simulink model "LKAS_AutoSave_DF_20220407_0926_SW62"  (R2018b)
settings: Solver=FixedStepDiscrete  StartTime=0.0  StopTime=10.0  FixedStep=0.01  RelTol=1e-3
InitFcn:
  | tmpVer = ver('MATLAB');
  | tmpVer = str2num(tmpVer.Version);
  | % -------------------------------------------------------------------
  | %  MATLAB file generated by Simulink.saveVars on 21-Nov-2019 10:06:14
  | %  MATLAB version: 7.13.0.564 (R2011b)
  | % -------------------------------------------------------------------
  | 
  | 
  | SInt16 = Simulink.AliasType;
  | SInt16.Description = 'Num';
  | if (tmpVer > 7.11)
  | 	SInt16.DataScope = 'Auto';
  | end
  | SInt16.HeaderFile = 'Rte_Type.h';
  | SInt16.BaseType = 'int16';
  | 
  | SInt32 = Simulink.AliasType;
  | SInt32.Description = 'Num';
  | if (tmpVer > 7.11)
  | 	SInt32.DataScope = 'Auto';
  | end
  | SInt32.HeaderFile = 'Rte_Type.h';
  | SInt32.BaseType = 'int32';
  | 
  | SInt8 = Simulink.AliasType;
  | SInt8.Description = 'Num';
  | if (tmpVer > 7.11)
  | 	SInt8.DataScope = 'Auto';
  | end
  | SInt8.HeaderFile = 'Rte_Type.h';
  | SInt8.BaseType = 'int8';
  | 
  | T_A_m2_1024_1_u32 = Simulink.NumericType;
  | T_A_m2_1024_1_u32.Description = 'm2 (square meters  (m2))';
  | if (tmpVer > 7.11)
  | 	T_A_m2_1024_1_u32.DataScope = 'Auto';
  | end
  | T_A_m2_1024_1_u32.HeaderFile = 'Rte_Type.h';
  | T_A_m2_1024_1_u32.DataTypeMode = 'Fixed-point: slope and bias scaling';
  | T_A_m2_1024_1_u32.SignednessBool = false;
  | T_A_m2_1024_1_u32.WordLength = 32;
  | T_A_m2_1024_1_u32.FixedExponent = -10;
  | T_A_m2_1024_1_u32.SlopeAdjustmentFactor = 1;
  | T_A_m2_1024_1_u32.Bias = 0;
  | T_A_m2_1024_1_u32.DataTypeOverride = 'Inherit';
  | T_A_m2_1024_1_u32.IsAlias = true;
  | 
  | T_A_m2_65536_1_u16 = Simulink.NumericType;
  | T_A_m2_65536_1_u16.Description = 'm2 (square meters  (m2))';
  | if (tmpVer > 7.11)
  | 	T_A_m2_65536_1_u16.DataScope = 'Auto';
  | end
  | T_A_m2_65536_1_u16.HeaderFile = 'Rte_Type.h';
  | T_A_m2_65536_1_u16.DataTypeMode = 'Fixed-point: slope and bias scaling';
  | T_A_m2_65536_1_u16.SignednessBool = false;
  | T_A_m2_65536_1_u16.WordLength = 16;
  | T_A_m2_65536_1_u16.FixedExponent = -16;
  | T_A_m2_65536_1_u16.SlopeAdjustmentFactor = 1;
  | T_A_m2_65536_1_u16.Bias = 0;
  | T_A_m2_65536_1_u16.DataTypeOverride = 'Inherit';
  | ... (+4664 lines)
StopFcn:
  | clear  T_A_m2_1024_1_u32 T_A_m2_65536_1_u16 T_A_m2_Float32 T_A_mm2_10_1_u16 T_A_mm2_4_1_s16 T_A_mm2_Float32 T_Cnt_Num_10_1_u32 T_Cnt_Num_1_1_s16 T_Cnt_Num_1_1_s32 T_Cnt_Num_1_1_s8 T_Cnt_Num_1_1_u16 T_Cnt_Num_1_1_u32 T_Cnt_Num_1_1_u8 T_E_J_1_1_s32 T_E_J_Float32 T_E_kJ_128_1_s32 T_E_kJ_Float32 T_E_kwh_10_1_u16 T_E_kwh_Float32 T_Epl_kwhpkm_100_1_u16 T_Epl_kwhpkm_Float32 T_F_N_1_1_s16 T_F_N_Float32 T_I_A_1000_1_u16 T_I_A_1048576_1_s32 T_I_A_2048_1_s16 T_I_A_32_1_s16 T_I_A_Float32 T_I_mA_1_1_s16 T_I_mA_32768_128_s16 T_I_mA_Float32 T_J_kgpm2_128_1_u16 T_J_kgpm2_Float32 T_K_NA_1000_1_s16 T_K_NA_100_1_s16 T_K_NA_100_1_u16 T_K_NA_1024_1_s16 T_K_NA_1024_1_u16 T_K_NA_128_1_s16 T_K_NA_128_1_u16 T_K_NA_128_1_u8 T_K_NA_16777216_1_u32 T_K_NA_16_1_s16 T_K_NA_16_1_u16 T_K_NA_16_1_u8 T_K_NA_1_16_u16 T_K_NA_1_1_s16 T_K_NA_1_1_u16 T_K_NA_1_1_u8 T_K_NA_32768_1_s16 T_K_NA_32768_1_u16 T_K_NA_32_1_s8 T_K_NA_4096_1_u16 T_K_NA_4194304_1_s32 T_K_NA_4194304_1_u16 T_K_NA_65536_1_s32 T_K_NA_65536_1_u16 T_K_NA_8192_1_s16 T_K_NA_8_1_s16 T_K_NA_Float32 T_M_Nm_16_1_s16 T_M_Nm_1_1_s16 T_M_Nm_32768_1_s16 T_M_Nm_32_1_s16 T_M_Nm_4_1_s16 T_M_Nm_512_1_s16 T_M_Nm_Float32 T_P_W_1_4_s16 T_P_W_1_8_s16 T_P_W_Float32 T_P_kW_128_1_s16 T_P_kW_1_8_s16 T_P_kW_8_1_s32 T_P_kW_Float32 T_Pct_pct_1024_1_s32 T_Pct_pct_1024_1_u32 T_Pct_pct_10_1_s16 T_Pct_pct_10_1_u32 T_Pct_pct_128_100_s8 T_Pct_pct_1_1_s16 T_Pct_pct_1_4_u8 T_Pct_pct_255_100_u16 T_Pct_pct_255_100_u8 T_Pct_pct_256_1_s16 T_Pct_pct_256_1_u16 T_Pct_pct_65535_100_u16 T_Pct_pct_Float32 T_R_ohm_1024_1_s16 T_R_ohm_32_1_s16 T_R_ohm_Float32 T_TK_K_16_1_s16 T_TK_K_Float32 T_T_degC_10_400_1_u16 T_T_degC_16_1_s16 T_T_degC_1_40_1_u8 T_T_degC_2_80_1_u8 T_T_degC_Float32 T_U_V_1000_1_u16 T_U_V_10_1_u8 T_U_V_200_1_u8 T_U_V_32_1_s16 T_U_V_4096_1_s16 T_U_V_512_1_s16 T_U_V_65535_8_u16 T_U_V_8192_1_u16 T_U_V_Float32 T_U_mV_1_1_s16 T_U_mV_256_20_u16 T_U_mV_Float32 T_V_l_256_1_s16 T_V_l_4096_1_s16 T_V_l_64_1_s16 T_V_l_65535_100_u16 T_V_l_Float32 T_V_ml_128_1_s16 T_V_ml_1_1_s16 T_V_ml_32768_1_s16 T_V_ml_Float32 T_V_ul_32_1_u16 T_V_ul_Float32 T_Vpl_clpkm_512_1_u16 T_Vpl_clpkm_Float32 T_a_kphps_16_1_s16 T_a_kphps_Float32 T_a_mps2_128_1_s16 T_a_mps2_Float32 T_c_MJpkg_256_1_s16 T_c_MJpkg_Float32 T_c_kJpgpK_1024_1_s16 T_c_kJpgpK_Float32 T_c_kJpkgpK_128_1_u16 T_c_kJpkgpK_Float32 T_chrg_Ah_1_1_s16 T_chrg_Ah_1_1_u16 T_chrg_Ah_1_1_u8 T_chrg_Ah_256_1_u16 T_chrg_Ah_4194304_1_s32 T_chrg_Ah_512_1_u16 T_chrg_Ah_8_1_u16 T_chrg_Ah_Float32 T_cmp_NA_100_1_s16 T_cmp_NA_128_1_s16 T_cmp_NA_16_1_s16 T_cmp_NA_32768_1_u16 T_cmp_NA_Float32 T_d2n_rpmps2_4_1_s16 T_d2n_rpmps2_Float32 T_dPct_pctps_16_1_s16 T_dPct_pctps_256_1_s16 T_dPct_pctps_Float32 T_dT_degCps_128_1_s16 T_dT_degCps_Float32 T_dV_lph_1_1_s16 T_dV_lph_Float32 T_dV_lpm_128_1_s16 T_dV_lpm_32_1_s16 T_dV_lpm_Float32 T_dV_lps_1024_1_u16 T_dV_lps_4_1_u16 T_dV_lps_Float32 T_dV_mlps_1024_1_s16 T_dV_mlps_Float32 T_d_BitField16 T_dm_gps_128_1_s16 T_dm_gps_128_1_u16 T_dm_gps_256_1_u16 T_dm_gps_Float32 T_dm_mgps_1_1_s16 T_dm_mgps_Float32 T_dn_rpmps_1_1_s16 T_dn_rpmps_2_1_s16 T_dn_rpmps_Float32 T_dp_Paps_1_1_s16 T_dp_Paps_Float32 T_dp_kPaps_1_1_s16 T_dp_kPaps_8_1_s16 T_dp_kPaps_Float32 T_dphi_degps_128_1_s16 T_dphi_degps_8_1_s16 T_dphi_degps_Float32 T_dr_ps_256_1_s16 T_dr_ps_Float32 T_drho_mgplps_1_2_s16 T_drho_mgplps_Float32 T_e_NA_1_1_u8 T_f_Hz_1_1_u16 T_f_Hz_1_1_u32 T_f_Hz_64_1_u16 T_f_Hz_8_1_s16 T_f_Hz_Float32 T_g_BitField32 T_l_km_16_1_s16 T_l_km_1_1_u16 T_l_km_1_1_u32 T_l_km_Float32 T_l_m_1024_1_s16 T_l_m_16_1_s16 T_l_m_1_1_u32 T_l_m_Float32 T_l_mm_16_1_s16 T_l_mm_1_1_u16 T_l_mm_4096_1_s16 T_l_mm_4_1_u8 T_l_mm_64_1_s16 T_l_mm_Float32 T_m_g_1_1_s16 T_m_g_2048_1_s16 T_m_g_32_1_u16 T_m_g_Float32 T_m_kg_1024_1_s16 T_m_kg_1_1_s16 T_m_kg_1_1_u32 T_m_kg_Float32 T_m_mg_128_1_s16 T_m_mg_32_1_s16 T_m_mg_Float32 T_n_rpm_1_1_s16 T_n_rpm_1_25_u8 T_n_rpm_256_50_u16 T_n_rpm_2_25_u8 T_n_rpm_4_1_u16 T_n_rpm_Float32 T_p_MPa_64_1_s16 T_p_MPa_Float32 T_p_Pa_1_1_s16 T_p_Pa_Float32 T_p_kPa_1_10_u16 T_p_kPa_1_1_s16 T_p_kPa_1_1_u8 T_p_kPa_256_1_u16 T_p_kPa_32_1_u16 T_p_kPa_64_1_s16 T_p_kPa_Float32 T_phi_deg_100_1_s16 T_phi_deg_1024_1_s16 T_phi_deg_128_1_s16 T_phi_deg_1_1_u8 T_phi_deg_256_1_s16 T_phi_deg_2_1_s8 T_phi_deg_32_1_s16 T_phi_deg_512_6_s32 T_phi_deg_Float32 T_phi_rad_2048_1_s16 T_phi_rad_Float32 T_r_NA_1024_1_s16 T_r_NA_1024_1_u16 T_r_NA_16384_1_s16 T_r_NA_16_1_s16 T_r_NA_256_1_s8 T_r_NA_256_1_u16 T_r_NA_32768_1_u16 T_r_NA_32_1_u16 T_r_NA_4096_1_s16 T_r_NA_65535_2_u16 T_r_NA_8192_1_u16 T_r_NA_Float32 T_rho_gpl_8192_1_s16 T_rho_gpl_Float32 T_rho_kgpm3_16_1_s16 T_rho_kgpm3_Float32 T_rho_mgpl_1_1_s16 T_rho_mgpl_64_1_s16 T_rho_mgpl_Float32 T_t_hour_1_1_s16 T_t_hour_Float32 T_t_m_1_1_u16 T_t_m_Float32 T_t_ms_1_1_s16 T_t_ms_1_1_u16 T_t_ms_1_1_u32 T_t_ms_4096_1_s16 T_t_ms_64_1_s16 T_t_ms_Float32 T_t_s_1000_1_s16 T_t_s_100_1_s16 T_t_s_10_1_s16 T_t_s_10_1_u16 T_t_s_1_1_s16 T_t_s_1_1_u16 T_t_s_1_1_u32 T_t_s_Float32 T_t_us_10_1_u32 T_t_us_1_1_s16 T_t_us_1_1_u32 T_t_us_1_4_u16 T_t_us_Float32 T_v_kph_1_1_u8 T_v_kph_64_1_s16 T_v_kph_64_1_u16 T_v_kph_Float32 T_v_mps_256_1_s16 T_v_mps_Float32 T_w_radps_32_1_s16 T_w_radps_Float32 T_y_BitField8 T_y_BitFieldDiagProgress T_y_BitFieldDiagStatus T_y_NA_1_1_u8 SInt16 SInt32 SInt8 T_BOOLEAN UInt16 UInt32 UInt8 s16 s32 s8 u16 u32 u8
model workspace (MAT data in the model file):
  MCOS : class17 (value not decoded)
  MCOS : class17 (value not decoded)
  MCOS : class17 (value not decoded)
  MCOS : class17 (value not decoded)
  MCOS : class17 (value not decoded)
  MCOS : class17 (value not decoded)
  MCOS : class17 (value not decoded)
  MCOS : class17 (value not decoded)
  MCOS : class17 (value not decoded)
  MCOS : class17 (value not decoded)
  MCOS : class17 (value not decoded)
  MCOS : class17 (value not decoded)
  MCOS : class17 (value not decoded)
  MCOS : class17 (value not decoded)
  MCOS : class17 (value not decoded)
  MCOS : class17 (value not decoded)
  MCOS : class17 (value not decoded)
  MCOS : class17 (value not decoded)
  MCOS : class17 (value not decoded)
  MCOS : class17 (value not decoded)
  MCOS : class17 (value not decoded)
  MCOS : class17 (value not decoded)
  MCOS : class17 (value not decoded)
  MCOS : class17 (value not decoded)
  MCOS : class17 (value not decoded)
  MCOS : class17 (value not decoded)
  MCOS : class17 (value not decoded)
  MCOS : class17 (value not decoded)
  MCOS : class17 (value not decoded)
  MCOS : class17 (value not decoded)
  MCOS : class17 (value not decoded)
  MCOS : class17 (value not decoded)
  MCOS : class17 (value not decoded)
  MCOS : class17 (value not decoded)
  MCOS : class17 (value not decoded)
  MCOS : class17 (value not decoded)
  MCOS : class17 (value not decoded)
  MCOS : class17 (value not decoded)
  MCOS : class17 (value not decoded)
  MCOS : class17 (value not decoded)
  MCOS : class17 (value not decoded)
  MCOS : class17 (value not decoded)
  MCOS : class17 (value not decoded)
  MCOS : class17 (value not decoded)
  MCOS : class17 (value not decoded)
  MCOS : class17 (value not decoded)
  MCOS : class17 (value not decoded)
  MCOS : class17 (value not decoded)
  MCOS : class17 (value not decoded)
  MCOS : class17 (value not decoded)
  MCOS : class17 (value not decoded)
  MCOS : class17 (value not decoded)
  MCOS : class17 (value not decoded)
  MCOS : class17 (value not decoded)
  MCOS : class17 (value not decoded)
  MCOS : class17 (value not decoded)
  MCOS : class17 (value not decoded)
  MCOS : class17 (value not decoded)
  MCOS : class17 (value not decoded)
  MCOS : class17 (value not decoded)
  MCOS : class17 (value not decoded)
  MCOS : class17 (value not decoded)
  MCOS : class17 (value not decoded)
  MCOS : class17 (value not decoded)
  MCOS : class17 (value not decoded)
  MCOS : class17 (value not decoded)
  MCOS : class17 (value not decoded)
  MCOS : class17 (value not decoded)
  MCOS : class17 (value not decoded)
  MCOS : class17 (value not decoded)
  MCOS : class17 (value not decoded)
  MCOS : class17 (value not decoded)
  MCOS : class17 (value not decoded)
  MCOS : class17 (value not decoded)
  MCOS : class17 (value not decoded)
  MCOS : class17 (value not decoded)
  MCOS : class17 (value not decoded)
  MCOS : class17 (value not decoded)
  MCOS : class17 (value not decoded)
  MCOS : class17 (value not decoded)
  MCOS : class17 (value not decoded)
  MCOS : class17 (value not decoded)
  MCOS : class17 (value not decoded)
  MCOS : class17 (value not decoded)
  MCOS : class17 (value not decoded)
  MCOS : class17 (value not decoded)
  MCOS : class17 (value not decoded)
  MCOS : class17 (value not decoded)
  MCOS : class17 (value not decoded)
  MCOS : class17 (value not decoded)
  MCOS : class17 (value not decoded)
  MCOS : class17 (value not decoded)
  MCOS : class17 (value not decoded)
  MCOS : class17 (value not decoded)
  MCOS : class17 (value not decoded)
  MCOS : class17 (value not decoded)
  MCOS : class17 (value not decoded)
  MCOS : class17 (value not decoded)
  MCOS : class17 (value not decoded)
  MCOS : class17 (value not decoded)
  MCOS : class17 (value not decoded)
  MCOS : class17 (value not decoded)
  MCOS : class17 (value not decoded)
  MCOS : class17 (value not decoded)
  MCOS : class17 (value not decoded)
  MCOS : class17 (value not decoded)
undefined symbols (not defined in the file): LKA_CarWidth, LKA_SampleTime, LKA_StrRatio_C, LKA_Veh2CamL_C, LKA_Veh2CamW_C, LKA_WhlBaseL_C, LL_CompHdAg_C, LL_CompSWA_C, LL_CrvtPrvwT_C, LL_DesDvt_C, LL_DvtComp_C, LL_DvtPrvwT_C, LL_DvtSpdDet_vDvtSpdMin_C, LL_HandsOff_ExitTime, LL_HandsOff_TextTime, LL_HandsOff_WarnTime, LL_HdAgExT_C, LL_HdAgPrvwT_C, LL_LAccMax_C, LL_LAccRMax_C, LL_LDW_EarliestWarnLine_C, LL_LDW_LatestWarnLine_C, LL_LDWS_SUPPRESS_HEADING, LL_LFClb_TFC_FfCtlRatio_C, LL_LFClb_TFC_KdBalance_C, LL_LFClb_TFC_KdMaxSWA_C, LL_LFClb_TFC_KdV1_C, LL_LFClb_TFC_KdV2_C, LL_LFClb_TFC_KdVehSpdLwr_C, LL_LFClb_TFC_KdVehSpdUpr_C, LL_LFClb_TFC_Ki_C, LL_LFClb_TFC_KiMaxSWA_C, LL_LFClb_TFC_Kp_C, LL_LFClb_TFC_KpKlat_C, LL_LFClb_TFC_KpV1_C, LL_LFClb_TFC_KpV2_C, LL_LFClb_TFC_KpVehSpdLwr_C, LL_LFClb_TFC_KpVehSpdUpr_C, LL_LFClb_TFC_PrvwT_C, LL_LKA_EarliestWarnLine_C, LL_LKA_LatestWarnLine_C, LL_LKAExPrcs_ExitC0Dvt, LL_LKAExPrcs_ExitC0Swt, LL_LKAExPrcs_tiExitDelayTime3, LL_LKAExPrcs_tiExitTime1, LL_LKAExPrcs_tiExitTime2, LL_LKAExPrcs_tiExitTime3, LL_LKAS_OUT_OF_CONTROL_LAT_VEL, LL_LKAS_OUT_OF_CONTROL_TTLC, LL_LKASWASyn_M0, LL_LKASWASyn_M1, LL_LKASWASyn_M2, LL_LKASWASyn_M3D, LL_LKASWASyn_M3K_DT, LL_LKASWASyn_M3K_MSD, LL_LKASWASyn_M4K, LL_LKASWASyn_SWAaddMax, LL_LKASWASyn_T2, LL_LKASWASyn_tiTrqSwaRtTime, LL_LKASWASyn_tiTrqSwaTime ... (+47)
libraries: simulink x234, canmsglib x6, dspstat3 x3, simulink_extras x1
(part 12 of 22)

== system LKAS_AutoSave_DF_20220407_0926_SW62/LKAS/LL/LLOn/LKA Input Processing (LKAInP)/Previewed Heading Angle Calculation (PrHdAg)/Perdicted Heading Angle from Right Lane Line (PrvwTTLCHdAgLftTTLCRgt) ==
  PrdcHdAgRgt_lPrvwDstZ : Inport
  PrdcHdAgRgt_bsR0Info : Inport  Port=2
  Add : Sum  Inputs=+++  AccumDataTypeStr=single
  Bus Selector : BusSelector  OutputSignals=R0_C1,R0_C2,R0_C3
  Gain : Gain  Gain=2  OutDataTypeStr=single
  Gain1 : Gain  Gain=3  OutDataTypeStr=single
  Product3 : Product  OutDataTypeStr=single  RndMeth=Zero
  Product4 : Product  OutDataTypeStr=single  RndMeth=Zero
  Z*Z : Product  OutDataTypeStr=single  RndMeth=Zero
  PrdcHdAgRgt_phiPrdcHdAgRgt : Outport
  wires:
  Add/1 -> PrdcHdAgRgt_phiPrdcHdAgRgt/1
  PrdcHdAgRgt_bsR0Info/1 -> Bus Selector/1
  PrdcHdAgRgt_lPrvwDstZ/1 -> Z*Z/1, Product3/2, Z*Z/2
  Bus Selector/1 -> Add/1  "<R0_C1>"
  Product3/1 -> Add/2
  Bus Selector/2 -> Gain/1  "<R0_C2>"
  Bus Selector/3 -> Gain1/1  "<R0_C3>"
  Product4/1 -> Add/3
  Z*Z/1 -> Product4/2
  Gain/1 -> Product3/1
  Gain1/1 -> Product4/1

== system LKAS_AutoSave_DF_20220407_0926_SW62/LKAS/LL/LLOn/LKA Input Processing (LKAInP)/Previewed Heading Angle Calculation (PrHdAg)/Perdicted Heading Angle from Right Lane Line (PrvwTTLCHdAgRgtTTLCRgt) ==
  PrdcHdAgRgt_lPrvwDstZ : Inport
  PrdcHdAgRgt_bsR0Info : Inport  Port=2
  Add : Sum  Inputs=+++  AccumDataTypeStr=single
  Bus Selector : BusSelector  OutputSignals=R0_C1,R0_C2,R0_C3
  Gain : Gain  Gain=2  OutDataTypeStr=single
  Gain1 : Gain  Gain=3  OutDataTypeStr=single
  Product3 : Product  OutDataTypeStr=single  RndMeth=Zero
  Product4 : Product  OutDataTypeStr=single  RndMeth=Zero
  Z*Z : Product  OutDataTypeStr=single  RndMeth=Zero
  PrdcHdAgRgt_phiPrdcHdAgRgt : Outport
  wires:
  Gain1/1 -> Product4/1
  Gain/1 -> Product3/1
  Z*Z/1 -> Product4/2
  Product4/1 -> Add/3
  Bus Selector/3 -> Gain1/1  "<R0_C3>"
  Bus Selector/2 -> Gain/1  "<R0_C2>"
  Product3/1 -> Add/2
  Bus Selector/1 -> Add/1  "<R0_C1>"
  PrdcHdAgRgt_lPrvwDstZ/1 -> Z*Z/2, Product3/2, Z*Z/1
  PrdcHdAgRgt_bsR0Info/1 -> Bus Selector/1
  Add/1 -> PrdcHdAgRgt_phiPrdcHdAgRgt/1

== system LKAS_AutoSave_DF_20220407_0926_SW62/LKAS/LL/LLOn/LKA Input Processing (LKAInP)/Previewed Heading Angle Calculation (PrHdAg)/Predicted Heading Angle from Left Lane Line (PrdcHdAgtLft)1 ==
  PrdcHdAgtLft_bsL0Info : Inport
  PrdcHdAgtLft_lPrvwDstZ : Inport  Port=2
  Add : Sum  Inputs=+++  AccumDataTypeStr=single
  Bus Selector : BusSelector  OutputSignals=L0_C1,L0_C2,L0_C3
  Gain : Gain  Gain=2  OutDataTypeStr=single
  Gain1 : Gain  Gain=3  OutDataTypeStr=single
  Product3 : Product  OutDataTypeStr=single  RndMeth=Zero
  Product4 : Product  OutDataTypeStr=single  RndMeth=Zero
  Z*Z : Product  OutDataTypeStr=single  RndMeth=Zero
  PrdcHdAgtLft_phiPrdcHdAgLft : Outport
  wires:
  Gain1/1 -> Product4/1
  Gain/1 -> Product3/1
  Z*Z/1 -> Product4/2
  Product4/1 -> Add/3
  Bus Selector/3 -> Gain1/1  "<L0_C3>"
  Bus Selector/2 -> Gain/1  "<L0_C2>"
  Product3/1 -> Add/2
  Bus Selector/1 -> Add/1  "<L0_C1>"
  PrdcHdAgtLft_lPrvwDstZ/1 -> Z*Z/2, Product3/2, Z*Z/1
  PrdcHdAgtLft_bsL0Info/1 -> Bus Selector/1
  Add/1 -> PrdcHdAgtLft_phiPrdcHdAgLft/1

== system LKAS_AutoSave_DF_20220407_0926_SW62/LKAS/LL/LLOn/LKA Input Processing (LKAInP)/Previewed Heading Angle Calculation (PrHdAg)/Predicted Heading Angle from Left Lane Line (PrdcHdAgtLftTTLCLft) ==
  PrdcHdAgtLft_bsL0Info : Inport
  PrdcHdAgtLft_lPrvwDstZ : Inport  Port=2
  Add : Sum  Inputs=+++  AccumDataTypeStr=single
  Bus Selector : BusSelector  OutputSignals=L0_C1,L0_C2,L0_C3
  Gain : Gain  Gain=2  OutDataTypeStr=single
  Gain1 : Gain  Gain=3  OutDataTypeStr=single
  Product3 : Product  OutDataTypeStr=single  RndMeth=Zero
  Product4 : Product  OutDataTypeStr=single  RndMeth=Zero
  Z*Z : Product  OutDataTypeStr=single  RndMeth=Zero
  PrdcHdAgtLft_phiPrdcHdAgLft : Outport
  wires:
  Gain1/1 -> Product4/1
  Gain/1 -> Product3/1
  Z*Z/1 -> Product4/2
  Product4/1 -> Add/3
  Bus Selector/3 -> Gain1/1  "<L0_C3>"
  Bus Selector/2 -> Gain/1  "<L0_C2>"
  Product3/1 -> Add/2
  Bus Selector/1 -> Add/1  "<L0_C1>"
  PrdcHdAgtLft_lPrvwDstZ/1 -> Z*Z/2, Product3/2, Z*Z/1
  PrdcHdAgtLft_bsL0Info/1 -> Bus Selector/1
  Add/1 -> PrdcHdAgtLft_phiPrdcHdAgLft/1

== system LKAS_AutoSave_DF_20220407_0926_SW62/LKAS/LL/LLOn/LKA Input Processing (LKAInP)/Previewed Heading Angle Calculation (PrHdAg)/Predicted Heading Angle from Left Lane Line (PrvwTTLCHdAgRgtTTLCLft) ==
  PrdcHdAgtLft_bsL0Info : Inport
  PrdcHdAgtLft_lPrvwDstZ : Inport  Port=2
  Add : Sum  Inputs=+++  AccumDataTypeStr=single
  Bus Selector : BusSelector  OutputSignals=L0_C1,L0_C2,L0_C3
  Gain : Gain  Gain=2  OutDataTypeStr=single
  Gain1 : Gain  Gain=3  OutDataTypeStr=single
  Product3 : Product  OutDataTypeStr=single  RndMeth=Zero
  Product4 : Product  OutDataTypeStr=single  RndMeth=Zero
  Z*Z : Product  OutDataTypeStr=single  RndMeth=Zero
  PrdcHdAgtLft_phiPrdcHdAgLft : Outport
  wires:
  Add/1 -> PrdcHdAgtLft_phiPrdcHdAgLft/1
  PrdcHdAgtLft_bsL0Info/1 -> Bus Selector/1
  PrdcHdAgtLft_lPrvwDstZ/1 -> Z*Z/1, Product3/2, Z*Z/2
  Bus Selector/1 -> Add/1  "<L0_C1>"
  Product3/1 -> Add/2
  Bus Selector/2 -> Gain/1  "<L0_C2>"
  Bus Selector/3 -> Gain1/1  "<L0_C3>"
  Product4/1 -> Add/3
  Z*Z/1 -> Product4/2
  Gain/1 -> Product3/1
  Gain1/1 -> Product4/1

== system LKAS_AutoSave_DF_20220407_0926_SW62/LKAS/LL/LLOn/LKA Input Processing (LKAInP)/Previewed Heading Angle Calculation (PrHdAg)/Z Calculation (ZCalc) ==
  ZCalc_vVehSpd : Inport
  ZCalc_tiHdAgPrvwT_C : Inport  Port=2
  Divide : Product  Inputs=**  OutDataTypeStr=single
  kph to mps : Gain  Gain=1/3.6  OutDataTypeStr=single
  ZCalc_lPrvwDstZ : Outport
  wires:
  kph to mps/1 -> Divide/1
  Divide/1 -> ZCalc_lPrvwDstZ/1
  ZCalc_tiHdAgPrvwT_C/1 -> Divide/2
  ZCalc_vVehSpd/1 -> kph to mps/1

== system LKAS_AutoSave_DF_20220407_0926_SW62/LKAS/LL/LLOn/LKA Input Processing (LKAInP)/Previewed Heading Angle Calculation (PrHdAg)/Z Calculation (ZCalc)1 ==
  ZCalc_vVehSpd : Inport
  ZCalc_tiHdAgPrvwT_C : Inport  Port=2
  Divide : Product  Inputs=**  OutDataTypeStr=single
  kph to mps : Gain  Gain=1/3.6  OutDataTypeStr=single
  ZCalc_lPrvwDstZ : Outport
  wires:
  kph to mps/1 -> Divide/1
  Divide/1 -> ZCalc_lPrvwDstZ/1
  ZCalc_tiHdAgPrvwT_C/1 -> Divide/2
  ZCalc_vVehSpd/1 -> kph to mps/1

== system LKAS_AutoSave_DF_20220407_0926_SW62/LKAS/LL/LLOn/LKA Input Processing (LKAInP)/Steering Wheel Position Calculation (SWAPosCal)/Subsystem ==
  SWAIn : Inport
  LKA_SampleTime : Inport  Port=2
  Enable : EnablePort
      settings: AttributesFormatString=states = %<StatesWhenEnabling>
  Constant : Constant  Value=10  OutDataTypeStr=single
  LowPass : Subsystem
  Saturation : Saturate  UpperLimit=3  LowerLimit=-3
      settings: AttributesFormatString="Min = %<LowerLimit>  Max = %<UpperLimit>"
  SWAPos : Outport  InitialOutput=0
      settings: AttributesFormatString=%<OutputWhenDisabled> = %<InitialOutput>
  wires:
  SWAIn/1 -> LowPass/2(u)
  LowPass/1(y) -> Saturation/1  "SWAPos"
  Constant/1 -> LowPass/1(T)
  LKA_SampleTime/1 -> LowPass/3(dT)
  Saturation/1 -> SWAPos/1

== system LKAS_AutoSave_DF_20220407_0926_SW62/LKAS/LL/LLOn/LKA Input Processing (LKAInP)/Steering Wheel Position Calculation (SWAPosCal)/Subsystem1 ==
  L0 : Inport
  R0 : Inport  Port=2
  VehSpd : Inport  Port=3
  SWA : Inport  Port=4
  LKA_SampleTime : Inport  Port=5
  Abs{2,4..7} (5 alike) : Abs
  Bus Selector : BusSelector  OutputSignals=L0_C1,L0_C2,L0_Q
  Bus Selector1 : BusSelector  OutputSignals=R0_C1,R0_C2,R0_Q
  Compare To Constant : simulink/Logic and Bit Operations/Compare To Constant  relop===  const=3.0  OutDataTypeStr=boolean
  Compare To Constant1 : simulink/Logic and Bit Operations/Compare To Constant  relop===  const=3.0  OutDataTypeStr=boolean
  Constant : Constant  Value=0.0001  OutDataTypeStr=single
  Constant1 : Constant  Value=0.008  OutDataTypeStr=single
  Constant3 : Constant  Value=2  OutDataTypeStr=single
  Constant4 : Constant  Value=35  OutDataTypeStr=single
  Constant5 : Constant  Value=4  OutDataTypeStr=single
  Divide : Product  Inputs=*/
  Logical Operator : Logic  AllPortsSameDT=off  OutDataTypeStr=boolean
  Logical Operator1 : Logic  AllPortsSameDT=off  OutDataTypeStr=boolean
  Logical Operator3 : Logic  Inputs=5  AllPortsSameDT=off  OutDataTypeStr=boolean
  Logical Operator4 : Logic  AllPortsSameDT=off  OutDataTypeStr=boolean
  Relational Operator{,1..3,7} (5 alike) : RelationalOperator  Operator=<=  OutDataTypeStr=boolean  RndMeth=Simplest
  Relational Operator6 : RelationalOperator  OutDataTypeStr=boolean  RndMeth=Simplest
  Subsystem : Subsystem
  Flg : Outport
  wires:
  L0/1 -> Bus Selector/1
  R0/1 -> Bus Selector1/1
  Logical Operator1/1 -> Logical Operator3/1
  Bus Selector/3 -> Compare To Constant/1  "<L0_Q>"
  Abs2/1 -> Relational Operator7/1
  Bus Selector1/3 -> Compare To Constant1/1  "<R0_Q>"
  Relational Operator2/1 -> Logical Operator1/1
  Compare To Constant1/1 -> Logical Operator4/2
  Relational Operator6/1 -> Logical Operator3/4
  Abs7/1 -> Relational Operator3/1
  Constant1/1 -> Relational Operator3/2, Relational Operator2/2
  Constant/1 -> Relational Operator1/2, Relational Operator/2
  Abs4/1 -> Relational Operator/1
  Constant3/1 -> Divide/1
  Logical Operator3/1 -> Subsystem/Enable, Subsystem/1(In)  "SWA"
  VehSpd/1 -> Relational Operator6/1
  Constant4/1 -> Relational Operator6/2
  Abs6/1 -> Relational Operator2/1
  Compare To Constant/1 -> Logical Operator4/1
  Relational Operator7/1 -> Logical Operator3/5
  Bus Selector1/2 -> Abs5/1  "<R0_C2>"
  Abs5/1 -> Relational Operator1/1
  Relational Operator1/1 -> Logical Operator/2
  Relational Operator3/1 -> Logical Operator1/2
  SWA/1 -> Abs2/1
  Logical Operator/1 -> Logical Operator3/2
  Constant5/1 -> Relational Operator7/2
  Subsystem/1(Out) -> Flg/1
  Bus Selector/1 -> Abs6/1  "<L0_C1>"
  Bus Selector1/1 -> Abs7/1  "<R0_C1>"
  Logical Operator4/1 -> Logical Operator3/3
  Bus Selector/2 -> Abs4/1  "<L0_C2>"
  Divide/1 -> Subsystem/2(In1)
  Relational Operator/1 -> Logical Operator/1
  LKA_SampleTime/1 -> Divide/2

== system LKAS_AutoSave_DF_20220407_0926_SW62/LKAS/LL/LLOn/LKA Input Processing (LKAInP)/Under The Limit (UndrLim)/Steering Wheel Angel Max (SWAMax) ==
  SWAMax_vVehSpd : Inport
  SWAMax_aLAcc_C : Inport  Port=2
  LKA_StrRatio_C : Inport  Port=3
  LKA_WhlBaseL_C : Inport  Port=4
  Constant : Constant  Value=0.09  OutDataTypeStr=single
  Divide1 : Product  Inputs=*/
  MATLAB Function : MATLAB Function  TreatAsAtomicUnit=on
  Saturation1 : Saturate  UpperLimit=0.0117  LowerLimit=0.00237
      settings: AttributesFormatString="Min = %<LowerLimit>  Max = %<UpperLimit>"
  Saturation3 : Saturate  UpperLimit=150  LowerLimit=60
      settings: AttributesFormatString="Min = %<LowerLimit>  Max = %<UpperLimit>"
  kph To mps : Gain  Gain=1/3.6  OutDataTypeStr=single
  SWAMax_phiSWAMax : Outport
  wires:
  LKA_StrRatio_C/1 -> MATLAB Function/3(i)
  LKA_WhlBaseL_C/1 -> MATLAB Function/4(L)
  kph To mps/1 -> MATLAB Function/1(v)
  SWAMax_vVehSpd/1 -> Saturation3/1, kph To mps/1
  Divide1/1 -> Saturation1/1
  Saturation1/1 -> MATLAB Function/5(K)
  SWAMax_aLAcc_C/1 -> MATLAB Function/2(ax)
  MATLAB Function/1(SWAmax) -> SWAMax_phiSWAMax/1
  Constant/1 -> Divide1/1
  Saturation3/1 -> Divide1/2  "Vx"

== system LKAS_AutoSave_DF_20220407_0926_SW62/LKAS/LL/LLOn/LKA Input Processing (LKAInP)/Under The Limit (UndrLim)/Steering Wheel Angel Rate Max (SWARMax) ==
  SWARateMax_vVehSpd : Inport
  SWARateMax_aLAccR_C : Inport  Port=2
  LKA_StrRatio_C : Inport  Port=3
  LKA_WhlBaseL_C : Inport  Port=4
  Constant : Constant  Value=0.09  OutDataTypeStr=single
  Divide1 : Product  Inputs=*/
  MATLAB Function : MATLAB Function  TreatAsAtomicUnit=on
  Saturation1 : Saturate  UpperLimit=0.0117  LowerLimit=0.00237
      settings: AttributesFormatString="Min = %<LowerLimit>  Max = %<UpperLimit>"
  Saturation3 : Saturate  UpperLimit=150  LowerLimit=60
      settings: AttributesFormatString="Min = %<LowerLimit>  Max = %<UpperLimit>"
  kph To mps : Gain  Gain=1/3.6  OutDataTypeStr=single
  SWARMax_dphiSWARMax : Outport
  wires:
  kph To mps/1 -> MATLAB Function/1(v)
  LKA_WhlBaseL_C/1 -> MATLAB Function/4(L)
  LKA_StrRatio_C/1 -> MATLAB Function/3(i)
  MATLAB Function/1(SWARmax) -> SWARMax_dphiSWARMax/1
  SWARateMax_vVehSpd/1 -> Saturation3/1, kph To mps/1
  Divide1/1 -> Saturation1/1
  Saturation1/1 -> MATLAB Function/5(K)
  SWARateMax_aLAccR_C/1 -> MATLAB Function/2(dax)
  Constant/1 -> Divide1/1
  Saturation3/1 -> Divide1/2  "Vx"

== system LKAS_AutoSave_DF_20220407_0926_SW62/LKAS/LL/LLOn/LL State Determination (LLStateDet)/LL State Machine Conditions (LLSMCon)/Activation Condition (ActvC) ==
  LKA_Mode : Inport
  bsInInfo : Inport  Port=2
  bsLKAInPInfo : Inport  Port=3
  bsLLClb : Inport  Port=4
  Activation Condition Synthesis (ActvCSyn) : Subsystem  Description=|
      | Block Name: Activation Condition Synthesis
      | Ab.: ActvCSyn
      | No.: 1.1.1.4.4
      | Rev: 0.0.1
      | Update Date: 19-3-26
  Bus Selector : BusSelector  OutputSignals=bsEPSInfo,bsLaneInfo.bsL0Info.L0_Q,bsLaneInfo.bsR0Info.R0_Q
  Bus Selector1 : BusSelector  OutputSignals=LaneWidth,bsDvtInfo.ILftDvt,bsDvtInfo.IRgtDvt
  Deviation Threshold Condition (DvtThresCon) : Subsystem
  EPS Controllability Enable Condition (EPSCtlEC) : Subsystem  Description=|
      | Block Name: EPS Controllability Enable Condition
      | Ab.: EPSCtlEC
      | No.: 1.1.1.4.1
      | Rev: 0.0.1
      | Update Date: 19-3-26
  Lane Quality Enable Condition (LaneQlEC) : Subsystem  Description=|
      | Block Name: Lane Quality Enable Condition
      | Ab.: LaneQlEC
      | No.: 1.1.1.4.3
      | Rev: 0.0.1
      | Update Date: 19-3-26
  stLDWActvCSyn : Outport
  stLKAActvCSyn : Outport  Port=2
  wires:
  bsInInfo/1 -> Bus Selector/1, Lane Quality Enable Condition (LaneQlEC)/1(LaneQlEC_InInfoSyn)
  Activation Condition Synthesis (ActvCSyn)/1(stLDWActvCSyn) -> stLDWActvCSyn/1  "stLDWActvCSyn"
  Deviation Threshold Condition (DvtThresCon)/2(stDvtThresActvFlgLKA) -> Activation Condition Synthesis (ActvCSyn)/4(stDvtThresActvFlgLKA), Lane Quality Enable Condition (LaneQlEC)/3(LaneQlEC_stDvtThresActvFlg)
  Bus Selector/1 -> EPS Controllability Enable Condition (EPSCtlEC)/1(EPSCtlEC_bsEPSInfo)  "<bsEPSInfo>"
  Bus Selector/2 -> Lane Quality Enable Condition (LaneQlEC)/4(LaneQlEC_stFacmL0Ql)  "<L0_Q>"
  Bus Selector/3 -> Lane Quality Enable Condition (LaneQlEC)/5(LaneQlEC_stFacmR0Ql)  "<R0_Q>"
  EPS Controllability Enable Condition (EPSCtlEC)/1(stEPSCtlEC) -> Activation Condition Synthesis (ActvCSyn)/2(stEPSCtlEC)
  Lane Quality Enable Condition (LaneQlEC)/1(stLaneQlECFlg) -> Activation Condition Synthesis (ActvCSyn)/5(stLaneQlECFlg)
  Activation Condition Synthesis (ActvCSyn)/2(stLKAActvCSyn) -> stLKAActvCSyn/1  "stLKAActvCSyn"
  bsLLClb/1 -> Deviation Threshold Condition (DvtThresCon)/4(DvtThresCon_bsDvtThresClb), Lane Quality Enable Condition (LaneQlEC)/2(LaneQlEC_SingleLane_Disable_Swt)
  Deviation Threshold Condition (DvtThresCon)/1(stDvtThresActvFlgLDW) -> Activation Condition Synthesis (ActvCSyn)/3(stDvtThresActvFlgLDW)
  bsLKAInPInfo/1 -> Bus Selector1/1, Deviation Threshold Condition (DvtThresCon)/5(DvtThresCon_LKAInfoSyn)
  Bus Selector1/2 -> Deviation Threshold Condition (DvtThresCon)/2(DvtThresCon_ILftDvt)  "<ILftDvt>"
  Bus Selector1/3 -> Deviation Threshold Condition (DvtThresCon)/3(DvtThresCon_IRgtDvt)  "<IRgtDvt>"
  Bus Selector1/1 -> Deviation Threshold Condition (DvtThresCon)/1(DvtThresCon_lLaneWidth)  "<LaneWidth>"
  LKA_Mode/1 -> [LKA_Mode]
  [LKA_Mode] -> Activation Condition Synthesis (ActvCSyn)/1(LKA_Mode)

== system LKAS_AutoSave_DF_20220407_0926_SW62/LKAS/LL/LLOn/LL State Determination (LLStateDet)/LL State Machine Conditions (LLSMCon)/Deactivation Condition (DeactvC) ==
  LKA_Mode : Inport
  bsInInfo : Inport  Port=2
  bsLKAInPInfo : Inport  Port=3
  bsLLClb : Inport  Port=4
  LLState : Inport  Port=5
  ExitFlg : Inport  Port=6
  Bus Selector : BusSelector  OutputSignals=bsVehMovInfo.ESC_VehSpd,bsEPSInfo
  Bus Selector1 : BusSelector  OutputSignals=LaneWidth,bsDvtInfo.ILftDvt,bsDvtInfo.IRgtDvt,bsPrCrvtInfo.crPrvwCrvt
  Deactivation Condition Synthesis (DeactvCSyn) : Subsystem  Description=|
      | Block Name: Deactivation Condition Synthesis
      | Ab.: DeactvCSyn
      | No.: 1.1.1.5.3
      | Rev: 0.0.1
      | Update Date: 19-3-26
  Deviation Threshold Condition (DvtThresCon) : Subsystem
  Driver Take Condition (DvrTkCon) : Subsystem  Description=|
      | Block Name: EPS Condition
      | Ab.: EPSC
      | No.: 1.1.1.5.2
      | Rev: 0.0.1
      | Update Date: 19-3-26
  EPS Condition (EPSC) : Subsystem  Description=|
      | Block Name: EPS Condition
      | Ab.: EPSC
      | No.: 1.1.1.5.2
      | Rev: 0.0.1
      | Update Date: 19-3-26
  stLDWDeactvCSyn : Outport
  stLKADeactvCSyn : Outport  Port=2
  wires:
  bsInInfo/1 -> Bus Selector/1
  Deactivation Condition Synthesis (DeactvCSyn)/1(stLDWDeactvCSyn) -> stLDWDeactvCSyn/1
  bsLLClb/1 -> Deviation Threshold Condition (DvtThresCon)/4(LLClb), Driver Take Condition (DvrTkCon)/3(LLClb), EPS Condition (EPSC)/1(LLClb)
  Deviation Threshold Condition (DvtThresCon)/2(stDvtThresActvFlgLKA) -> Deactivation Condition Synthesis (DeactvCSyn)/3(stDvtThresActvFlgLKA), Driver Take Condition (DvrTkCon)/2(DvtThresCon_stDvtThresActvFlgLKA)
  LLState/1 -> EPS Condition (EPSC)/3(LLState)
  Bus Selector/2 -> EPS Condition (EPSC)/2(bsEPSInfo), Driver Take Condition (DvrTkCon)/5(bsEPSInfo)  "<bsEPSInfo>"
  EPS Condition (EPSC)/1(EPSC_stEPSCFlg) -> Deactivation Condition Synthesis (DeactvCSyn)/5(EPSC_stEPSCFlg)
  ExitFlg/1 -> Deactivation Condition Synthesis (DeactvCSyn)/6(ExitFlg)
  LKA_Mode/1 -> Deactivation Condition Synthesis (DeactvCSyn)/1(LKAMode)
  Deactivation Condition Synthesis (DeactvCSyn)/2(stLKADeactvCSyn) -> stLKADeactvCSyn/1  "stLKADeactvCSyn"
  Bus Selector/1 -> Driver Take Condition (DvrTkCon)/4(ESC_VehSpd)  "<ESC_VehSpd>"
  Driver Take Condition (DvrTkCon)/1(stDvrTkConFlg) -> Deactivation Condition Synthesis (DeactvCSyn)/4(stDvrTkConFlg)
  bsLKAInPInfo/1 -> Deviation Threshold Condition (DvtThresCon)/5(LKAInPInfo), Bus Selector1/1
  Bus Selector1/3 -> Deviation Threshold Condition (DvtThresCon)/3(IRgtDvt)  "<IRgtDvt>"
  Bus Selector1/2 -> Deviation Threshold Condition (DvtThresCon)/2(ILftDvt)  "<ILftDvt>"
  Bus Selector1/4 -> Driver Take Condition (DvrTkCon)/1(crPrvwCrvt)  "<crPrvwCrvt>"
  Bus Selector1/1 -> Deviation Threshold Condition (DvtThresCon)/1(LaneWidth)  "<LaneWidth>"
  Deviation Threshold Condition (DvtThresCon)/1(stDvtThresActvFlgLDW) -> Deactivation Condition Synthesis (DeactvCSyn)/2(stDvtThresActvFlgLDW)

== system LKAS_AutoSave_DF_20220407_0926_SW62/LKAS/LL/LLOn/LL State Determination (LLStateDet)/LL State Machine Conditions (LLSMCon)/Disable Condition (DisblC) ==
  LKA_Mode : Inport
  bsInInfo : Inport  Port=2
  bsLKAInPInfo : Inport  Port=3
  bsLLClb : Inport  Port=4
  LLState : Inport  Port=5
  Disable Condition Synthesis (DisblCSyn) : Subsystem  Description=|
      | Block Name: Disable Condition Synthesis
      | Ab.: DisblCSyn
      | No.: 1.1.1.3.8.0
      | Rev: 0.0.1
      | Update Date: 19-3-26
  Driver Intent Condition (DrvInttC) : Subsystem  Description=|
      | Block Name: Driver Intent Condition
      | Ab.: DrvInttC
      | No.: 1.1.1.3.3.0
      | Rev: 0.0.1
      | Update Date: 19-3-26
  LDW Alarm Timeout (LDWAlrmTOut) : Subsystem  Description=|
      | Block Name: LDW Alarm Timeout
      | Ab.: LDWAlrmTOut
      | No.: 1.1.1.3.6.0
      | Rev: 0.0.1
      | Update Date: 19-3-26
  LDW Own Condition (LDWOwnC) : Subsystem  Description=|
      | Block Name: LDW Own Condition
      | Ab.: LDWOwnC
      | No.: 1.1.1.3.4.0
      | Rev: 0.0.1
      | Update Date: 19-3-26
  LKA Own Condition (LKAOwnC) : Subsystem  Description=|
      | Block Name: LKA Own Condition
      | Ab.: LKAOwnC
      | No.: 1.1.1.3.5.0
      | Rev: 0.0.1
      | Update Date: 19-3-26
  Lane Condition (LaneC) : Subsystem  Description=|
      | Block Name: Lane Condition
      | Ab.: LaneC
      | No.: 1.1.1.3.2.0
      | Rev: 0.0.1
      | Update Date: 19-3-26
  Subsystem : Subsystem  Commented=on
  Subsystem1 : Subsystem
  Vehicle State Condition (VehStateC) : Subsystem  Description=|
      | Block Name: Vehicle State Condition
      | Ab.: VehStateC
      | No.: 1.1.1.3.1.0
      | Rev: 0.0.1
      | Update Date: 19-3-26
  stLDWDisblCSyn : Outport
  stLKADisblCSyn : Outport  Port=2
  Disable_Reason : Outport  Port=3
  wires:
  Vehicle State Condition (VehStateC)/1(stVehStateC) -> [stVehStateC]  "stVehStateC"
  LDW Own Condition (LDWOwnC)/1(stLDWOwnC) -> [stLDWOwnC]  "stLDWOwnC"
  Disable Condition Synthesis (DisblCSyn)/1(stLDWDisblCSyn) -> stLDWDisblCSyn/1  "stLDWDisblCSyn"
  LDW Alarm Timeout (LDWAlrmTOut)/1(stLDWAlrmTOut) -> [stLDWAlrmTOut]  "stLDWAlrmTOut"
  Disable Condition Synthesis (DisblCSyn)/2(stLKADisblCSyn) -> stLKADisblCSyn/1  "stLKADisblCSyn"
  LKA Own Condition (LKAOwnC)/2(LKAOwnCSyn) -> [LKAOwnCSyn]  "LKAOwnCSyn"
  Driver Intent Condition (DrvInttC)/2(DrvInttCSyn) -> [DrvInttCSyn]  "DrvInttCSyn"
  Lane Condition (LaneC)/2(LaneCSyn) -> [LaneCSyn]  "LaneCSyn"
  Vehicle State Condition (VehStateC)/2(VehStateC) -> [VehStateC]  "VehStateC"
  Subsystem1/1(DisableReason) -> Disable_Reason/1  "Disable_Reason"
  LKA_Mode/1 -> [LKA_Mode]
  [LKA_Mode] -> Disable Condition Synthesis (DisblCSyn)/1(LKA_Mode)  "LKA_Mode"
  [LKA_Mode] -> Vehicle State Condition (VehStateC)/1(LKA_Mode)  "LKA_Mode"
  [LKA_Mode] -> LDW Own Condition (LDWOwnC)/1(LKA_Mode)  "LKA_Mode"
  [LKA_Mode] -> LKA Own Condition (LKAOwnC)/1(LKA_Mode)  "LKA_Mode"
  Lane Condition (LaneC)/1(stLaneC) -> [stLaneC]  "stLaneC"
  Driver Intent Condition (DrvInttC)/1(stDrvInttC) -> [stDrvInttC]  "stDrvInttC"
  LKA Own Condition (LKAOwnC)/1(stLKAOwnC) -> [stLKAOwnC]  "stLKAOwnC"
  [stVehStateC] -> Disable Condition Synthesis (DisblCSyn)/2(stVehStateC)
  [stLaneC] -> Disable Condition Synthesis (DisblCSyn)/3(stLaneC)
  [stDrvInttC] -> Disable Condition Synthesis (DisblCSyn)/4(stDrvInttC)
  [stLKAOwnC] -> Disable Condition Synthesis (DisblCSyn)/7(stLKAOwnC)
  [stLDWOwnC] -> Disable Condition Synthesis (DisblCSyn)/5(stLDWOwnC)
  [stLDWAlrmTOut] -> Disable Condition Synthesis (DisblCSyn)/6(stLDWAlrmTOut)
  LDW Alarm Timeout (LDWAlrmTOut)/2(LDWAlrmTOutSyn) -> [LDWAlrmTOutSyn]  "LDWAlrmTOutSyn"
  [LDWAlrmTOutSyn] -> Subsystem1/6(LDWAlrmTOut)
  [DrvInttCSyn] -> Subsystem1/3(DrvInttCSyn)
  [LDWOwnCSyn] -> Subsystem1/4(LDWOwnCSyn)
  [LKAOwnCSyn] -> Subsystem1/5(LKAOwnCSyn)
  [LaneCSyn] -> Subsystem1/2(LaneCSyn)
  [VehStateC] -> Subsystem1/1(VehStateC)
  bsLLClb/1 -> [LLClb]
  [LLClb] -> Vehicle State Condition (VehStateC)/3(LLClb)  "LLClb"
  [LLClb] -> Lane Condition (LaneC)/3(LLClb)  "LLClb"
  [LLClb] -> Driver Intent Condition (DrvInttC)/2(DrvInttC_bsLLClb)  "LLClb"
  [LLClb] -> LDW Own Condition (LDWOwnC)/3(LLClb)  "LLClb"
  [LLClb] -> LKA Own Condition (LKAOwnC)/5(LLClb)  "LLClb"
  [LLClb] -> LDW Alarm Timeout (LDWAlrmTOut)/2(LDWAlrmTOut_bsLLClb)
  LLState/1 -> [LLState]
  [LLState] -> Vehicle State Condition (VehStateC)/4(LLState)  "LLState"
  [LLState] -> LKA Own Condition (LKAOwnC)/4(LLState)  "LLState"
  [LLState] -> LDW Alarm Timeout (LDWAlrmTOut)/1(LDWAlrmTOut_bsLLState)
  bsInInfo/1 -> [InInfoSyn]
  [InInfoSyn] -> Vehicle State Condition (VehStateC)/2(InInfoSyn)  "InInfoSyn"
  [InInfoSyn] -> Lane Condition (LaneC)/1(InInfoSyn)  "InInfoSyn"
  [InInfoSyn] -> Driver Intent Condition (DrvInttC)/1(DrvInttC_bsInInfoSyn)  "InInfoSyn"
  [InInfoSyn] -> LKA Own Condition (LKAOwnC)/2(InInfoSyn)  "InInfoSyn"
  bsLKAInPInfo/1 -> [LKAInPInfo]
  [LKAInPInfo] -> Lane Condition (LaneC)/2(LKAInPInfo)  "LKAInPInfo"
  [LKAInPInfo] -> Driver Intent Condition (DrvInttC)/3(LKAInPInfo)  "LKAInPInfo"
  [LKAInPInfo] -> LDW Own Condition (LDWOwnC)/2(LKAInPInfo)  "LKAInPInfo"
  [LKAInPInfo] -> LKA Own Condition (LKAOwnC)/3(LKAInPInfo)  "LKAInPInfo"
  LDW Own Condition (LDWOwnC)/2(LDWOwnCSyn) -> [LDWOwnCSyn]  "LDWOwnCSyn"

== system LKAS_AutoSave_DF_20220407_0926_SW62/LKAS/LL/LLOn/LL State Determination (LLStateDet)/LL State Machine Conditions (LLSMCon)/Enable Condition (EnaC) ==
  LKA_Mode : Inport
  bsInInfo : Inport  Port=2
  bsLKAInPInfo : Inport  Port=3
  bsLLClb : Inport  Port=4
  Driver Intent Condition (DrvInttC) : Subsystem  Description=|
      | Block Name: Driver Intent Condition
      | Ab.: DrvInttC
      | No.: 1.1.1.2.3.0
      | Rev: 0.0.1
      | Update Date: 19-3-26
  Enable Condition Synthesis (EnaCSyn) : Subsystem  Description=|
      | Block Name: Enable Condition Synthesis
      | Ab.: EnaCSyn
      | No.: 1.1.1.2.7.0
      | Rev: 0.0.1
      | Update Date: 19-3-26
  LDW Own Condition (LDWOwnC) : Subsystem  Description=|
      | Block Name: LDW Own Condition
      | Ab.: LDWOwnC
      | No.: 1.1.1.2.4.0
      | Rev: 0.0.1
      | Update Date: 19-3-26
  LKA Own Condition (LKAOwnC) : Subsystem  Description=|
      | Block Name: LKA Own Condition
      | Ab.: LKAOwnC
      | No.: 1.1.1.2.5.0
      | Rev: 0.0.1
      | Update Date: 19-3-26
  Lane Condition (LaneC) : Subsystem  Description=|
      | Block Name: Lane Condition
      | Ab.: LaneC
      | No.: 1.1.1.2.2.0
      | Rev: 0.0.1
      | Update Date: 19-3-26
  Vehicle State Condition (VehStateC) : Subsystem  Description=|
      | Block Name: Vehicle State Condition
      | Ab.: VehStateC
      | No.: 1.1.1.2.1.0
      | Rev: 0.0.1
      | Update Date: 19-3-26
  stLDWEnaCSyn : Outport
  stLKAEnaCSyn : Outport  Port=2
  wires:
  Enable Condition Synthesis (EnaCSyn)/1(stLDWEnaCSyn) -> stLDWEnaCSyn/1  "stLDWEnaCSyn"
  LKA_Mode/1 -> [LKA_Mode]
  Enable Condition Synthesis (EnaCSyn)/2(stLKAEnaCSyn) -> stLKAEnaCSyn/1  "stLKAEnaCSyn"
  [LKA_Mode] -> Enable Condition Synthesis (EnaCSyn)/1(LKA_Mode)  "LKA_Mode"
  [LKA_Mode] -> Vehicle State Condition (VehStateC)/1(LKA_Mode)
  [stVehStateC] -> Enable Condition Synthesis (EnaCSyn)/2(stVehStateC)
  [stLaneC] -> Enable Condition Synthesis (EnaCSyn)/3(stLaneC)
  [stDrvInttC] -> Enable Condition Synthesis (EnaCSyn)/4(stDrvInttC)
  [stLKAOwnC] -> Enable Condition Synthesis (EnaCSyn)/6(stLKAOwnC)
  [stLDWOwnC] -> Enable Condition Synthesis (EnaCSyn)/5(stLDWOwnC)
  Vehicle State Condition (VehStateC)/1(stVehStateC) -> [stVehStateC]
  Lane Condition (LaneC)/1(stLaneC) -> [stLaneC]  "stLaneC"
  Driver Intent Condition (DrvInttC)/1(stDrvInttC) -> [stDrvInttC]  "stDrvInttC"
  LDW Own Condition (LDWOwnC)/1(stLDWOwnC) -> [stLDWOwnC]  "stLDWOwnC"
  LKA Own Condition (LKAOwnC)/1(stLKAOwnC) -> [stLKAOwnC]  "stLKAOwnC"
  bsInInfo/1 -> [InInfoSyn]  "InInfoSyn"
  bsLKAInPInfo/1 -> [LKAInPInfo]  "LKAInPInfo"
  bsLLClb/1 -> [LLClb]  "LLClb"
  [InInfoSyn] -> Vehicle State Condition (VehStateC)/2(InInfoSyn)
  [InInfoSyn] -> Lane Condition (LaneC)/1(InInfoSyn)
  [InInfoSyn] -> Driver Intent Condition (DrvInttC)/1(InInfoSyn)
  [InInfoSyn] -> LKA Own Condition (LKAOwnC)/2(InInfoSyn)
  [LLClb] -> Vehicle State Condition (VehStateC)/3(LLClb)
  [LLClb] -> Lane Condition (LaneC)/3(LLClb)
  [LLClb] -> Driver Intent Condition (DrvInttC)/2(LLClb)
  [LLClb] -> LDW Own Condition (LDWOwnC)/3(LLClb)
  [LLClb] -> LKA Own Condition (LKAOwnC)/4(LLClb)
  [LKAInPInfo] -> Lane Condition (LaneC)/2(LKAInPInfo)
  [LKA_Mode] -> LDW Own Condition (LDWOwnC)/1(LKA_Mode)
  [LKAInPInfo] -> LDW Own Condition (LDWOwnC)/2(LKAInPInfo)
  [LKAInPInfo] -> LKA Own Condition (LKAOwnC)/3(LKAInPInfo)
  [LKA_Mode] -> LKA Own Condition (LKAOwnC)/1(LKA_Mode)

== system LKAS_AutoSave_DF_20220407_0926_SW62/LKAS/LL/LLOn/LL State Determination (LLStateDet)/LL State Machine Conditions (LLSMCon)/Fault Condition (FaultC) ==
  note: 52:轮速信号/轮速脉冲错误
  note: 54:SAS故障状态
  note: 82:转向灯开关异常
  note: 124:EPS 方向盘转角信号无效或超出范围,连续三次故障
  note: 125:整车CAN上方向盘扭矩信号无效，连续三次故障
  note: 126:EPS/LKA握手信号无效或超出范围,连续三次故障
  note: 127:车速信号无效或超出范围，连续三次故障
  note: 130:横向加速度信号无效或超出范围,连续三次故障
  note: 131:纵向加速度信号无效或超出范围,连续三次故障
  note: 139:LKA模式信号超出范围，连续三次故障
  note: 142:方向盘转角信号无效或超出范围，连续三次故障
  note: 143:方向盘转速信号无效，连续三次故障
  note: 145:实际档位信号无效或超出范围，连续三次故障
  note: 148:连续三次检测到前摄像头状态异常
  note: 电池电压超出范围
  note: BSW\ASW诊断结果已经在ADIA中经过开机后5s判断
  FaultC_bsInInfoSyn : Inport
  FaultC_bsLLClb : Inport  Port=2
  FaultC_SignalFault : Inport  Port=3
  16Bits_Set2 : Subsystem
  AND : Logic  AllPortsSameDT=off  OutDataTypeStr=boolean
  Bus Selector1 : BusSelector  OutputSignals=bsBSWFaultStatus.ADIAve_e_Node_EPS_Validity,bsBSWFaultStatus.ADIAve_e_Node_ESC_Validity,bsBSWFaultStatus.ADIAve_e_Node_IBCM_Validity,bsBSWFaultStatus.ADIAve_e_Node_SAS_Validity,bsBSWFaultStatus.ADIAve_e_Node_IC_Validity,bsBSWFaultStatus.ADIAve_e_Node_MP5_Validity,bsBSWFaultStatus.ADIAve_e_Node_TCU_Validity
  Bus Selector2 : BusSelector  OutputSignals=bsEPSInfo.EPS_LKA_State
  Bus Selector4 : BusSelector  OutputSignals=bsASWFaultStatus.ADIA_DTC_WheelSpdFaultSignal,bsASWFaultStatus.ADIA_DTC_SAS_SASFailureSts,bsASWFaultStatus.ADIA_DTC_BCM_TurnSwFailure,bsASWFaultStatus.ADIA_DTC_EPS2_17A_InvOorSteAngle,bsASWFaultStatus.ADIA_DTC_EPS2_17A_InvStTorq,bsASWFaultStatus.ADIA_DTC_EPS3_31C_InvOorLKAState,bsASWFaultStatus.ADIA_DTC_ESC2_A0_InvOorVehSpeed,bsASWFaultStatus.ADIA_DTC_ESC5_122_InvOorLongiAccel,bsASWFaultStatus.ADIA_DTC_ESC5_122_InvOorLatAccel,bsASWFaultStatus.ADIA_DTC_GW_MP5_413_OorLKAMode,bsASWFaultStatus.ADIA_DTC_SAS_A5_InvOorSteAngle,bsASWFaultStatus.ADIA_DTC_SAS_A5_InvRotSpeed,bsASWFaultStatus.ADIA_DTC_TCU1_93_InvOorGear,bsASWFaultStatus.ADIA_DTC_CameraSystemError,bsASWFaultStatus.ADIA_DTC_BatteryOutOfRange
  Bus Selector5 : BusSelector  OutputSignals=bsConstantClb.LKA_SampleTime
  Bus Selector6 : BusSelector  OutputSignals=bsASWFaultStatus.ADIA_DTC_WheelSpdFaultSignal,bsASWFaultStatus.ADIA_DTC_SAS_SASFailureSts,bsASWFaultStatus.ADIA_DTC_BCM_TurnSwFailure,bsASWFaultStatus.ADIA_DTC_EPS2_17A_InvOorSteAngle,bsASWFaultStatus.ADIA_DTC_EPS2_17A_InvStTorq,bsASWFaultStatus.ADIA_DTC_EPS3_31C_InvOorLKAState,bsASWFaultStatus.ADIA_DTC_ESC2_A0_InvOorVehSpeed,bsASWFaultStatus.ADIA_DTC_ESC5_122_InvOorLongiAccel,bsASWFaultStatus.ADIA_DTC_ESC5_122_InvOorLatAccel,bsASWFaultStatus.ADIA_DTC_GW_MP5_413_OorLKAMode,bsASWFaultStatus.ADIA_DTC_SAS_A5_InvOorSteAngle,bsASWFaultStatus.ADIA_DTC_SAS_A5_InvRotSpeed,bsASWFaultStatus.ADIA_DTC_TCU1_93_InvOorGear,bsASWFaultStatus.ADIA_DTC_CameraSystemError,bsASWFaultStatus.ADIA_DTC_BatteryOutOfRange
  Bus Selector7 : BusSelector  OutputSignals=bsBSWFaultStatus.ADIAve_e_Node_EPS_Validity,bsBSWFaultStatus.ADIAve_e_Node_ESC_Validity,bsBSWFaultStatus.ADIAve_e_Node_IBCM_Validity,bsBSWFaultStatus.ADIAve_e_Node_SAS_Validity,bsBSWFaultStatus.ADIAve_e_Node_IC_Validity,bsBSWFaultStatus.ADIAve_e_Node_MP5_Validity,bsBSWFaultStatus.ADIAve_e_Node_TCU_Validity
  Compare To Constant14 : simulink/Logic and Bit Operations/Compare To Constant  relop===  const=4  OutDataTypeStr=boolean
  Count_5s1 : Subsystem
  Ground{,1..10} (11 alike) : Ground
  Logical Operator1 : Logic  Operator=OR  Inputs=15  AllPortsSameDT=off  OutDataTypeStr=boolean
  Logical Operator10 : Logic  Operator=OR  AllPortsSameDT=off  OutDataTypeStr=boolean
  Logical Operator2 : Logic  Operator=OR  Inputs=7  AllPortsSameDT=off  OutDataTypeStr=boolean
  Logical Operator8 : Logic  Operator=OR  Inputs=3  AllPortsSameDT=off  OutDataTypeStr=boolean
  FaultC_stLDWFaultCSyn : Outport
  FaultC_stLKAFaultCSyn : Outport  Port=2
  Fault_Reason : Outport  Port=3
  wires:
  Ground10/1 -> 16Bits_Set2/20(Bit19)
  Compare To Constant14/1 -> AND/1  "EPS_State_For_LKA_Fault"
  AND/1 -> Logical Operator8/3  "EPS_Fault"
  Logical Operator8/1 -> [LKA_Fault], FaultC_stLKAFaultCSyn/1  "LKA_Fault"
  Logical Operator10/1 -> [LDW_Fault], FaultC_stLDWFaultCSyn/1  "LDW_Fault"
  FaultC_bsInInfoSyn/1 -> Bus Selector2/1
  Bus Selector2/1 -> Compare To Constant14/1  "<EPS_LKA_State>"
  FaultC_bsLLClb/1 -> Bus Selector5/1
  [BSW_Diagnostic] -> Logical Operator8/1, Logical Operator10/1  "CAN_Bus_Fault"
  Bus Selector5/1 -> [SampleTime]  "<LKA_SampleTime>"
  [SampleTime] -> Count_5s1/1(SampleTime)
  Bus Selector6/1 -> Logical Operator1/1  "<ADIA_DTC_WheelSpdFaultSignal>"
  Bus Selector6/2 -> Logical Operator1/2  "<ADIA_DTC_SAS_SASFailureSts>"
  Bus Selector1/1 -> Logical Operator2/1  "<ADIAve_e_Node_EPS_Validity>"
  FaultC_SignalFault/1 -> Bus Selector1/1, Bus Selector7/1, Bus Selector4/1, Bus Selector6/1
  Bus Selector6/3 -> Logical Operator1/3  "<ADIA_DTC_BCM_TurnSwFailure>"
  Bus Selector6/4 -> Logical Operator1/4  "<ADIA_DTC_EPS2_17A_InvOorSteAngle>"
  Bus Selector6/5 -> Logical Operator1/5  "<ADIA_DTC_EPS2_17A_InvStTorq>"
  Bus Selector6/6 -> ?  "<ADIA_DTC_EPS3_31C_InvOorLKAState>"
  Bus Selector6/8 -> ?  "<ADIA_DTC_ESC5_122_InvOorLongiAccel>"
  Bus Selector6/9 -> ?  "<ADIA_DTC_ESC5_122_InvOorLatAccel>"
  Bus Selector6/10 -> Logical Operator1/10  "<ADIA_DTC_GW_MP5_413_OorLKAMode>"
  Bus Selector6/13 -> ?  "<ADIA_DTC_TCU1_93_InvOorGear>"
  Bus Selector6/14 -> Logical Operator1/14  "<ADIA_DTC_CameraSystemError>"
  Bus Selector6/15 -> Logical Operator1/15  "<ADIA_DTC_BatteryOutOfRange>"
  Bus Selector6/7 -> Logical Operator1/7  "<ADIA_DTC_ESC2_A0_InvOorVehSpeed>"
  Bus Selector6/11 -> ?  "<ADIA_DTC_SAS_A5_InvOorSteAngle>"
  Bus Selector6/12 -> Logical Operator1/12  "<ADIA_DTC_SAS_A5_InvRotSpeed>"
  Bus Selector1/2 -> Logical Operator2/2  "<ADIAve_e_Node_ESC_Validity>"
  Bus Selector1/3 -> Logical Operator2/3  "<ADIAve_e_Node_IBCM_Validity>"
  Bus Selector1/4 -> Logical Operator2/4  "<ADIAve_e_Node_SAS_Validity>"
  Bus Selector1/5 -> ?  "<ADIAve_e_Node_IC_Validity>"
  Bus Selector1/6 -> Logical Operator2/6  "<ADIAve_e_Node_MP5_Validity>"
  Bus Selector1/7 -> Logical Operator2/7  "<ADIAve_e_Node_TCU_Validity>"
  Logical Operator1/1 -> [ASW_Diagnostic]  "ASW_Diagnostic"
  Logical Operator2/1 -> [BSW_Diagnostic]  "BSW_Diagnostic"
  Count_5s1/1(Out) -> AND/2  "Count_5s1"
  [ASW_Diagnostic] -> Logical Operator10/2, Logical Operator8/2  "Signal_Fault"
  Ground/1 -> Logical Operator1/6
  Bus Selector4/1 -> 16Bits_Set2/1(Bit0)  "<ADIA_DTC_WheelSpdFaultSignal>"
  Bus Selector4/2 -> 16Bits_Set2/2(Bit1)  "<ADIA_DTC_SAS_SASFailureSts>"
  Bus Selector4/3 -> 16Bits_Set2/3(Bit2)  "<ADIA_DTC_BCM_TurnSwFailure>"
  Bus Selector4/4 -> 16Bits_Set2/4(Bit3)  "<ADIA_DTC_EPS2_17A_InvOorSteAngle>"
  Bus Selector4/5 -> 16Bits_Set2/5(Bit4)  "<ADIA_DTC_EPS2_17A_InvStTorq>"
  Bus Selector4/6 -> 16Bits_Set2/6(Bit5)  "<ADIA_DTC_EPS3_31C_InvOorLKAState>"
  Bus Selector4/7 -> 16Bits_Set2/7(Bit6)  "<ADIA_DTC_ESC2_A0_InvOorVehSpeed>"
  Bus Selector4/8 -> ?  "<ADIA_DTC_ESC5_122_InvOorLongiAccel>"
  Bus Selector4/9 -> ?  "<ADIA_DTC_ESC5_122_InvOorLatAccel>"
  Bus Selector4/10 -> 16Bits_Set2/10(Bit9)  "<ADIA_DTC_GW_MP5_413_OorLKAMode>"
  Bus Selector4/11 -> ?  "<ADIA_DTC_SAS_A5_InvOorSteAngle>"
  Bus Selector4/12 -> 16Bits_Set2/12(Bit11)  "<ADIA_DTC_SAS_A5_InvRotSpeed>"
  Bus Selector4/13 -> ?  "<ADIA_DTC_TCU1_93_InvOorGear>"
  Bus Selector4/14 -> 16Bits_Set2/14(Bit13)  "<ADIA_DTC_CameraSystemError>"
  Bus Selector4/15 -> 16Bits_Set2/15(Bit14)  "<ADIA_DTC_BatteryOutOfRange>"
  16Bits_Set2/1(Index_32Bits) -> Fault_Reason/1  "Fault_Reason"
  Bus Selector7/1 -> 16Bits_Set2/16(Bit15)  "<ADIAve_e_Node_EPS_Validity>"
  Bus Selector7/2 -> 16Bits_Set2/17(Bit16)  "<ADIAve_e_Node_ESC_Validity>"
  Bus Selector7/3 -> 16Bits_Set2/18(Bit17)  "<ADIAve_e_Node_IBCM_Validity>"
  Bus Selector7/4 -> 16Bits_Set2/19(Bit18)  "<ADIAve_e_Node_SAS_Validity>"
  Bus Selector7/5 -> ?  "<ADIAve_e_Node_IC_Validity>"
  Bus Selector7/6 -> 16Bits_Set2/21(Bit20)  "<ADIAve_e_Node_MP5_Validity>"
  Bus Selector7/7 -> 16Bits_Set2/22(Bit21)  "<ADIAve_e_Node_TCU_Validity>"
  [LDW_Fault] -> 16Bits_Set2/23(Bit22)
  [LKA_Fault] -> 16Bits_Set2/24(Bit23)
  Ground1/1 -> Logical Operator1/8
  Ground2/1 -> Logical Operator1/9
  Ground3/1 -> 16Bits_Set2/8(Bit7)
  Ground4/1 -> 16Bits_Set2/9(Bit8)
  Ground5/1 -> Logical Operator1/11
  Ground6/1 -> 16Bits_Set2/11(Bit10)
  Ground8/1 -> 16Bits_Set2/13(Bit12)
  Ground7/1 -> Logical Operator1/13
  Ground9/1 -> Logical Operator2/5

== system LKAS_AutoSave_DF_20220407_0926_SW62/LKAS/LL/LL Inputs Mapping/bsLaneInfo/LanesReconstruct /RoadSide Offset/HdAgCompL0C1 ==
  LL_CompHdAg_C : Inport
  L0_Q : Inport  Port=2
  L0_C1 : Inport  Port=3
  Add : Sum
  Compare To Constant1 : simulink/Logic and Bit Operations/Compare To Constant  relop===  const=3  OutDataTypeStr=boolean
  Switch1 : Switch  Criteria=u2 > Threshold
  Out1 : Outport
  wires:
  Add/1 -> Switch1/1
  L0_C1/1 -> Add/2, Switch1/3
  LL_CompHdAg_C/1 -> Add/1
  Switch1/1 -> Out1/1  "L0_C1"
  L0_Q/1 -> Compare To Constant1/1
  Compare To Constant1/1 -> Switch1/2
